simulink model "ROCR6II_URDF_file"  (R2020b)
settings: Solver=FixedStepAuto  StartTime=0.0  StopTime=500  FixedStep=0.5  RelTol=1e-3
values from neighbouring files (symbols this model uses):
  X = [x,y,z,Roll,Pitch,Yaw]    [T2RPY.m]
undefined symbols (not defined in the file or in its folder): Y, Z
libraries: sm_lib x75, nesl_utility x7
(part 3 of 3)

== matlab function ROCR6II_URDF_file/impedent_control/MATLAB Function1 ==
  data: q input; M output
function M = M_num(q)
%M_NUM
%    M = M_NUM(Q1,Q2,Q3,Q4,Q5,Q6)
q1=q(1);q2=q(2);q3=q(3);q4=q(4);q5=q(5);q6=q(6);
%    This function was generated by the Symbolic Math Toolbox version 8.6.
%    07-Dec-2021 16:24:19

t2 = cos(q1);
t3 = cos(q2);
t4 = cos(q3);
t5 = cos(q4);
t6 = cos(q5);
t7 = cos(q6);
t8 = sin(q1);
t9 = sin(q2);
t10 = sin(q3);
t11 = sin(q4);
t12 = sin(q5);
t13 = sin(q6);
t14 = q2+q3;
t15 = q2+q5;
t16 = q3+q4;
t17 = q2.*2.0;
t18 = q3.*2.0;
t19 = q4.*2.0;
t20 = q5.*2.0;
t21 = q6.*2.0;
t33 = -q5;
t22 = t6.^2;
t23 = t7.^2;
t24 = sin(t20);
t25 = cos(t14);
t26 = cos(t15);
t27 = cos(t16);
t28 = q4+t14;
t29 = q5+t14;
t30 = sin(t14);
t31 = sin(t15);
t32 = sin(t16);
t34 = -t20;
t35 = -t21;
t36 = t2.*t6;
t39 = t2.*t12;
t40 = t6.*t8;
t44 = t8.*t12;
t45 = q2+t14;
t49 = q2+t33;
t50 = t14.*2.0;
t52 = t14+t33;
t64 = t6.*(3.9e+1./4.0e+2);
t65 = t5.*(5.7e+1./5.0e+2);
t66 = t11.*(5.7e+1./5.0e+2);
t83 = t5.*t12.*(3.9e+1./4.0e+2);
t84 = t11.*t12.*(3.9e+1./4.0e+2);
t99 = t4.*1.014787488e-1;
t121 = t6.*2.10083e-2;
t122 = t12.*2.10083e-2;
t125 = t6.*1.5925e-4;
t127 = t6.*8.86e-5;
t128 = t12.*8.86e-5;
t129 = t7.*t12.*t13.*1.889999999999997e-6;
t132 = t11.*1.114986e-1;
t136 = t5.*1.114986e-1;
t140 = t10.*2.65188e-5;
t146 = t5.*7.16878548e-5;
t152 = t5.*3.58439274e-5;
t163 = t11.*t12.*3.58439274e-5;
t164 = t4.*t5.*t6.*3.99274128e-5;
t165 = t4.*t11.*t12.*3.99274128e-5;
t166 = t5.*t10.*t12.*3.99274128e-5;
t167 = t6.*t10.*t11.*3.99274128e-5;
t169 = t5.*t12.*4.4321768397e-3;
t170 = t5.*t12.*8.8643536794e-3;
t171 = t6.*t11.*4.4321768397e-3;
t176 = t4.*t5.*t12.*4.9371083784e-3;
t177 = t4.*t6.*t11.*4.9371083784e-3;
t178 = t5.*t6.*t10.*4.9371083784e-3;
t179 = t10.*t11.*t12.*4.9371083784e-3;
t184 = t11.*8.27276665554e-2;
t197 = t11.*4.13638332777e-2;
t202 = t4.*t11.*5.55435170928e-2;
t203 = t5.*t10.*5.55435170928e-2;
t222 = t3.*1.5989248968e-5;
t225 = t9.*5.962436486703985e-3;
t230 = t12.*9.06307056372e-6;
t234 = t6.*1.94303003751466e-3;
t37 = cos(t28);
t38 = cos(t29);
t41 = q5+t28;
t42 = sin(t28);
t43 = sin(t29);
t46 = q2+t28;
t51 = cos(t49);
t53 = sin(t49);
t54 = t20+t28;
t57 = t14+t28;
t58 = cos(t52);
t59 = t28+t33;
t60 = t28+t34;
t61 = sin(t52);
t80 = -t66;
t82 = t19+t50;
t85 = -t83;
t93 = t64+1.065e-1;
t100 = t65+t84;
t123 = -t122;
t124 = t23.*1.889999999999997e-6;
t137 = -t132;
t147 = t31.*4.7336741892e-3;
t148 = t32.*9.4673483784e-3;
t149 = t26.*1.99637064e-5;
t150 = t27.*3.99274128e-5;
t151 = -t146;
t157 = t6.*t146;
t158 = -t152;
t161 = t6.*t152;
t175 = -t163;
t180 = -t165;
t181 = -t166;
t182 = -t167;
t185 = -t170;
t186 = -t169;
t187 = -t171;
t190 = t25.*1.6725731e-5;
t192 = -t176;
t193 = -t177;
t194 = -t178;
t196 = -t184;
t200 = -t197;
t206 = -t202;
t207 = -t203;
t214 = t30.*7.78686501734e-2;
t223 = t24.*9.27729949366e-6;
t240 = t121+t128-1.065e-1;
t252 = t22.*2.77326877791351e-3;
t277 = t129+t230+t234;
t47 = cos(t41);
t48 = sin(t41);
t55 = t7.*t37;
t56 = t13.*t37;
t62 = cos(t54);
t63 = sin(t54);
t67 = cos(t59);
t68 = cos(t60);
t69 = sin(t59);
t70 = sin(t60);
t71 = t36.*t37;
t72 = t37.*t39;
t73 = t37.*t40;
t74 = t2.*t7.*t42;
t75 = t6.*t7.*t42;
t76 = t37.*t44;
t77 = t2.*t13.*t42;
t78 = t7.*t8.*t42;
t79 = t6.*t13.*t42;
t81 = t8.*t13.*t42;
t101 = t2.*t93;
t102 = t8.*t93;
t106 = t66+t85;
t108 = t4.*t100;
t109 = t10.*t100;
t115 = t80+t83+2.37e+2./1.0e+3;
t126 = -t124;
t131 = t22.*t124;
t141 = t24.*t42.*7.962500000000001e-5;
t153 = -t147;
t154 = -t149;
t155 = -t150;
t159 = t53.*4.7336741892e-3;
t162 = t43.*4.24954841985e-3;
t168 = t38.*1.79219637e-5;
t173 = t51.*1.99637064e-5;
t195 = t61.*4.24954841985e-3;
t198 = -t190;
t201 = t58.*1.79219637e-5;
t224 = t123+t127;
t226 = -t223;
t238 = t42.*7.92876906372e-6;
t245 = t37.*1.663963245953534e-2;
t255 = -t252;
t298 = t175+t187+t277;
t86 = -t72;
t87 = -t73;
t88 = -t77;
t89 = -t78;
t90 = -t79;
t91 = t36+t76;
t92 = t44+t71;
t97 = t56+t75;
t107 = -t102;
t110 = t4.*t106;
t111 = t10.*t106;
t112 = -t109;
t118 = t4.*t115;
t119 = t10.*t115;
t130 = t56.*9.296e-5;
t133 = t75.*9.296e-5;
t134 = t55.*9.485e-5;
t135 = t47.*7.962500000000001e-5;
t138 = t79.*9.485e-5;
t139 = t67.*7.962500000000001e-5;
t144 = -t141;
t172 = -t159;
t174 = -t162;
t183 = -t168;
t188 = -t173;
t199 = -t195;
t205 = -t201;
t227 = t5.*t224;
t228 = t11.*t224;
t229 = t63.*4.63864974683e-6;
t231 = t47.*4.002781743233e-5;
t232 = t70.*4.63864974683e-6;
t237 = t48.*3.52200536814e-6;
t239 = t48.*1.258507593186e-5;
t241 = -t238;
t243 = t67.*3.85924222008233e-3;
t244 = t69.*3.52200536814e-6;
t248 = t69.*1.258507593186e-5;
t251 = t62.*2.911421944783775e-4;
t253 = t68.*2.911421944783775e-4;
t299 = t180+t181+t193+t194+t298;
t301 = t126+t131+t158+t161+t186+t200+t226+t255+3.08503415834179e-2;
t303 = t99+t126+t131+t140+t148+t151+t155+t157+t164+t179+t182+t185+t192+t196+t206+t207+t226+t255+3.379819209690679e-1;
t94 = t39+t87;
t95 = t40+t86;
t96 = t7.*t92;
t98 = t13.*t92;
t104 = t55+t90;
t113 = -t111;
t142 = -t138;
t143 = -t139;
t145 = t109+t110;
t204 = t108+t119;
t208 = t7.*t12.*t97.*9.296e-5;
t209 = t112+t118;
t210 = t12.*t42.*t91.*1.5925e-4;
t215 = -t9.*(t109-t118);
t233 = -t229;
t235 = -t231;
t236 = -t232;
t242 = t130+t133;
t246 = -t243;
t247 = -t244;
t254 = -t251;
t264 = t136+t228;
t272 = t137+t227+2.37e+2./1.0e+3;
t302 = t148+t155+t164+t179+t182+t192+t206+t207+t301;
t103 = t7.*t94;
t105 = t13.*t94;
t114 = t74+t98;
t116 = t88+t96;
t156 = t108+t113;
t160 = t9.*t145;
t211 = t3.*t204;
t212 = t9.*t204;
t213 = t12.*t42.*t95.*1.5925e-4;
t217 = t12.*t13.*t104.*9.485e-5;
t219 = t209+3.3e+1./1.25e+2;
t249 = t134+t142;
t250 = t135+t143;
t257 = -t242.*(t77-t96);
t259 = t242.*(t77-t96);
t267 = t4.*t264;
t268 = t10.*t264;
t273 = t4.*t272;
t274 = t10.*t272;
t117 = t81+t103;
t120 = t89+t105;
t189 = t3.*t156;
t191 = -t160;
t216 = -t212;
t218 = -t217;
t220 = t3.*t219;
t221 = t9.*t219;
t261 = t114.*t249;
t262 = t211+t215;
t263 = -t249.*(t78-t105);
t269 = -t268;
t278 = t267+t274;
t256 = t189+t191;
t258 = t117.*t242;
t265 = t211+t221;
t266 = t216+t220;
t270 = -t2.*(t212-t220);
t271 = -t8.*(t212-t220);
t280 = t9.*t278;
t281 = t8.*(t102+t2.*(t212-t220)).*(t160-t189).*(2.2e+1./1.25e+2);
t283 = t269+t273+3.3e+1./1.25e+2;
t287 = t8.*t262.*(t102+t2.*(t212-t220)).*(-2.2e+1./1.25e+2);
t288 = t8.*t262.*(t102+t2.*(t212-t220)).*(2.2e+1./1.25e+2);
t292 = t213+t259+t261;
t260 = -t258;
t275 = t101+t271;
t276 = t107+t270;
t282 = -t281;
t284 = t3.*t283;
t290 = t8.*t265.*(t102+t2.*(t212-t220)).*(-2.2e+1./1.25e+2);
t291 = t8.*t265.*(t102+t2.*(t212-t220)).*(2.2e+1./1.25e+2);
t294 = t8.*t292;
t296 = -t2.*(-t210+t258+t249.*(t78-t105));
t297 = t2.*(-t210+t258+t249.*(t78-t105));
t279 = t2.*t275.*(t160-t189).*(-2.2e+1./1.25e+2);
t285 = -t284;
t286 = t2.*t262.*t275.*(2.2e+1./1.25e+2);
t289 = t2.*t265.*t275.*(2.2e+1./1.25e+2);
t293 = t210+t260+t263;
t295 = -t294;
t300 = t280+t285;
M = reshape([t4.*(-1.63367952e-2)+t11.*8.4990968397e-3+t140+t148+t155+t158+cos(t17).*2.536047323340805e-1-cos(t45).*1.63367952e-2-cos(t46).*3.99274128e-5+cos(t50).*9.9389672074375e-2-cos(t57).*3.58439274e-5-cos(t82).*5.82284388956755e-4-sin(t17).*1.61248862826e-4+sin(t45).*2.65188e-5+sin(t46).*9.4673483784e-3+sin(t50).*2.88759272e-5+sin(t57).*8.4990968397e-3-sin(t82).*9.27729949366e-6+t12.^2.*t42.^2.*1.5925e-4+t97.*t242+t104.*t249+(t2.*t240+t8.*t300).^2.*1.707+(t8.*t240-t2.*t300).^2.*1.707+t37.*(t37.*1.975e-3+t6.*t42.*7.8e-6-t12.*t42.*9.92e-5)+(t102+t2.*(t212-t220)).^2.*(2.2e+1./1.25e+2)+t275.^2.*(2.2e+1./1.25e+2)+t12.*t42.*(t37.*(-9.92e-5)+t6.*t42.*6.1e-6+t12.*t42.*1.6808e-3)+t6.*t42.*(t37.*7.8e-6+t6.*t42.*2.092e-3+t12.*t42.*6.1e-6)+4.762913488144671e-1,t144+t149+t153+t168+t172+t174+t188+t198+t199+t205+t208+t214+t218+t222+t225+t233+t235+t236+t237+t241+t245+t246+t248+t253+t254+t289+t291,t144+t168+t174+t198+t199+t205+t208+t214+t218+t233+t235+t236+t237+t241+t245+t246+t248+t253+t254+t286+t288,t144+t208+t218+t233+t235+t236+t237+t241+t245+t246+t248+t253+t254+t279+t282,t37.*(-2.72839557767695e-3)+t47.*3.85924222008233e-3-t67.*4.002781743233e-5+t147+t154+t162+t172+t183+t188+t199+t205+t239+t247-t13.*t97.*9.296e-5-t7.*t104.*9.485e-5+(t39.*(3.9e+1./4.0e+2)-t73.*(3.9e+1./4.0e+2)).*(t102+t2.*(t212-t220)).*(2.2e+1./1.25e+2)-t275.*(t44.*(3.9e+1./4.0e+2)+t71.*(3.9e+1./4.0e+2)).*(2.2e+1./1.25e+2),t250,t149+t153+t168+t172+t174+t188+t198+t199+t205+t214+t222+t225+t233+t235+t236+t237+t241+t245+t246+t248+t253+t254+t289+t291+t295+t297,t4.*2.029574976e-1+t10.*5.30376e-5-t27.*7.98548256e-5+t32.*1.89346967568e-2+t126+t131+t151+t157+t185+t196+t226+t255-t4.*t11.*1.110870341856e-1-t5.*t10.*1.110870341856e-1+t4.*t5.*t6.*7.98548256e-5-t4.*t5.*t12.*9.874216756800001e-3-t6.*t10.*t11.*7.98548256e-5+t10.*t11.*t12.*9.874216756800001e-3+9.851289596233629e-1,t303,t302,t299,t125,t168+t174+t198+t199+t205+t214+t233+t235+t236+t237+t241+t245+t246+t248+t253+t254+t286+t288+t295+t297,t303,t126+t131+t151+t157+t185+t196+t226+t255+3.379819209690679e-1,t301,t298,t125,t233+t235+t236+t237+t241+t245+t246+t248+t253+t254+t279+t282+t295+t297,t302,t301,t126+t131+t226+t255+3.08503415834179e-2,t277,t125,t31.*2.4685541892e-3-t37.*4.49540057767695e-3+t43.*2.21608841985e-3+t47.*1.96735222008233e-3-t53.*2.4685541892e-3-t61.*2.21608841985e-3+t67.*2.432218256767e-5+t154+t183+t188+t205+t239+t247-cos(t21+t28).*4.724999999999993e-7-cos(t21+t41).*2.362499999999996e-7-cos(t28+t35).*4.724999999999993e-7+cos(t35+t41).*2.362499999999996e-7-cos(t21+t59).*2.362499999999996e-7+cos(t35+t59).*2.362499999999996e-7,t299,t298,t277,cos(t21).*9.449999999999986e-7+4.49540057767695e-3,0.0,t250,t125,t125,t125,0.0,1.5925e-4],[6,6]);

== matlab function ROCR6II_URDF_file/impedent_control/Subsystem/trToRPY1 ==
  data: T input; X output
function  X=Tr2Pos(T)
%#codegen
coder.extrinsic('disp'); %Declare disp as extrinsic
    %% 求末端位置
    x=T(1,4);y=T(2,4);z=T(3,4);
    %% 根据X-Y-Z固定角计算
    R=T;rpy=[0,0,0];
    if abs(abs(R(3,1)) - 1) < 0.000001  % when |R31| == 1
    % singularity
        rpy(1) = 0;     % roll is zero
        if R(3,1) < 0
            rpy(3) = -atan2(R(1,2), R(1,3));  % R-Y
        else
            rpy(3) = atan2(-R(1,2), -R(1,3));  % R+Y
        end
        rpy(2) = -asin(R(3,1));
    else
        rpy(1) = atan2(R(3,2), R(3,3));  % R
        rpy(3) = atan2(R(2,1), R(1,1));  % Y

        [~,k] = max(abs( [R(1,1) R(2,1) R(3,2) R(3,3)] ));
        switch k
            case 1
                rpy(2) = -atan(R(3,1)*cos(rpy(3))/R(1,1));
            case 2
                rpy(2) = -atan(R(3,1)*sin(rpy(3))/R(2,1));
            case 3
                rpy(2) = -atan(R(3,1)*sin(rpy(1))/R(3,2));
            case 4
                rpy(2) = -atan(R(3,1)*cos(rpy(1))/R(3,3));
        end
    end
%     RPY=rpy*180/pi;
    RPY=rpy;
    Roll=RPY(1);Pitch=RPY(2);Yaw=RPY(3);
    X=[x,y,z,Roll,Pitch,Yaw];
end

== matlab function ROCR6II_URDF_file/impedent_control/MATLAB Function5 ==
  data: Jana input; dx output; dq input
function dx = fcn(Jana,dq)
dx=Jana*dq;
end

== matlab function ROCR6II_URDF_file/impedent_control/acc->vel1 ==
  data: ddxe input; dxe input; dxe_targ output
function dxe_targ   = acc_integral(ddxe,dxe)
%% parameter
% dt = 0.001;
dt = 0.02;
dxe_targ=zeros(1,6);
dt_ddxe=ddxe*dt;
dxe_targ(1)=dxe(1)+dt_ddxe(1);
dxe_targ(2)=dxe(2)+dt_ddxe(2);
dxe_targ(3)=dxe(3)+dt_ddxe(3);
dxe_targ(4)=dxe(4)+dt_ddxe(4);
dxe_targ(5)=dxe(5)+dt_ddxe(5);
dxe_targ(6)=dxe(6)+dt_ddxe(6);
end

== matlab function ROCR6II_URDF_file/T1 ==
  data: q input; q output
function q = offset(q)
q(2) = q(2) + pi/2;
q(4) = q(4) + pi/2;

end

== matlab function ROCR6II_URDF_file/impedent_control/Subsystem/J_1 ==
  data: phi input; JaDown3 output; theta input; xi input; J input
function JaDown3 = Jana(phi,theta,xi,J)
om2eulmat=[cos(theta)*cos(xi), -sin(xi), 0;
    cos(theta)*sin(xi),  cos(xi), 0;
    -sin(theta),       0, 1];
omega=J(4:6,:);
JaDown3 = om2eulmat\omega;
end

== matlab function ROCR6II_URDF_file/impedent_control/vel->pos1 ==
  data: dxe input; xe input; xe_targ output
function xe_targ   = vel_integral(dxe,xe)
%% parameter
xe_targ=zeros(1,6);
% dt = 0.001;
dt = 0.02;
dt_dxe=dxe*dt;
xe_targ(1)=xe(1)+dt_dxe(1);
xe_targ(2)=xe(2)+dt_dxe(2);
xe_targ(3)=xe(3)+dt_dxe(3);
xe_targ(4)=xe(4)+dt_dxe(4);
xe_targ(5)=xe(5)+dt_dxe(5);
xe_targ(6)=xe(6)+dt_dxe(6);

end
